simulink subsystem "MovingCorrelation"  (R2022a)
settings: Solver=VariableStepAuto  StartTime=0.0  StopTime=10.0  RelTol=1e-3
libraries: simulink x2, dspstat3 x1
settings Model: Creator=targi  LastModifiedBy=targi

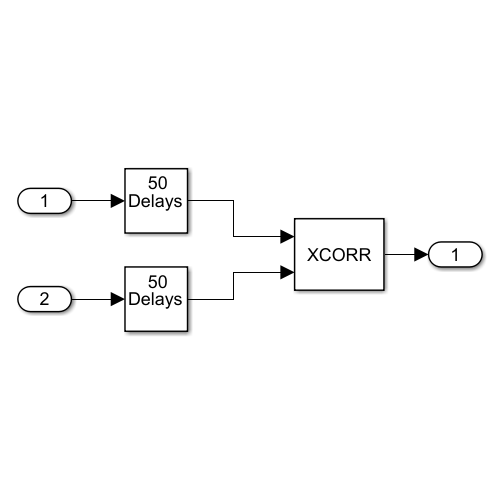
[thumbnail: Simulink's stored preview of the top-level diagram]
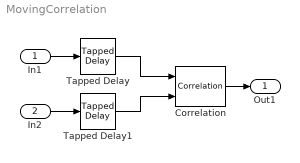
== system MovingCorrelation ==
  In1 : Inport
  In2 : Inport  Port=2
  Correlation : dspstat3/Correlation  domain=Time  roundingMode=Floor  overflowMode=off  outputDataTypeStr=Inherit: Same as accumulator  outputMin=[]  outputMax=[]  outputLastDataTypeStr=Inherit: Same as accumulator
      settings: SourceProductBaseCode=DS
  Tapped Delay : simulink/Discrete/Tapped Delay  vinit=0.0  samptime=-1  NumDelays=50  DelayOrder=Oldest  includeCurrent=off
  Tapped Delay1 : simulink/Discrete/Tapped Delay  vinit=0.0  samptime=-1  NumDelays=50  DelayOrder=Oldest  includeCurrent=off
  Out1 : Outport
  wires:
  Tapped Delay1/1 -> Correlation/2
  Tapped Delay/1 -> Correlation/1
  In2/1 -> Tapped Delay1/1
  In1/1 -> Tapped Delay/1
  Correlation/1 -> Out1/1
